simulink model "Kalman_filter"  (R2019b)
settings: Solver=FixedStepAuto  StartTime=0.0  StopTime=10.0  FixedStep=20e-3  RelTol=1e-3
values from neighbouring files (symbols this model uses):
  C = [0, 1]    [model_parameters.m]
undefined symbols (not defined in the file or in its folder): B_d, F, Q, R
settings Model: Creator=Олег  LastModifiedBy=Олег

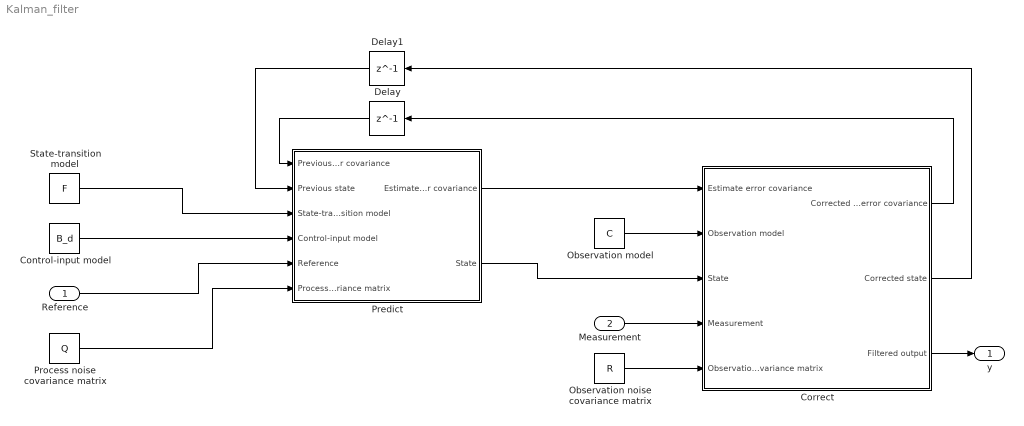
== system Kalman_filter ==
  Reference : Inport  PortDimensions=2
  Measurement : Inport  Port=2  PortDimensions=2
  Control-input model : Constant  Value=B_d
  Correct : Subsystem
  Delay : Delay  DelayLength=1  InitialCondition=eye(4)
  Delay1 : Delay  DelayLength=1  InitialCondition=zeros(4,1)
  Observation model : Constant  Value=C
  Observation noise covariance matrix : Constant  Value=R
  Predict : Subsystem
  Process noise covariance matrix : Constant  Value=Q
  State-transition model : Constant  Value=F
  y : Outport
  wires:
  State-transition model/1 -> Predict/3(State-transition model)
  Control-input model/1 -> Predict/4(Control-input model)
  Reference/1 -> Predict/5(Reference)
  Process noise covariance matrix/1 -> Predict/6(Process noise covariance matrix)
  Predict/2(State) -> Correct/3(State)
  Delay/1 -> Predict/1(Previous estimate error covariance)
  Delay1/1 -> Predict/2(Previous state)
  Predict/1(Estimate error covariance) -> Correct/1(Estimate error covariance)
  Observation model/1 -> Correct/2(Observation model)
  Measurement/1 -> Correct/4(Measurement)
  Observation noise covariance matrix/1 -> Correct/5(Observation noise covariance matrix)
  Correct/1(Corrected estimate error covariance) -> Delay/1
  Correct/2(Corrected state) -> Delay1/1
  Correct/3(Filtered output) -> y/1

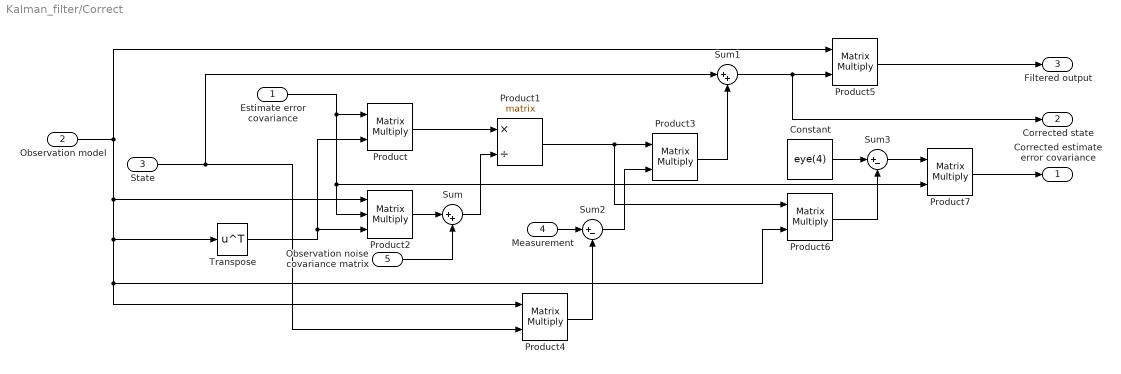
== system Kalman_filter/Correct ==
  Estimate error covariance : Inport
  Observation model : Inport  Port=2
  State : Inport  Port=3
  Measurement : Inport  Port=4
  Observation noise covariance matrix : Inport  Port=5
  Constant : Constant  Value=eye(4)
  Product{,3..7} (6 alike) : Product  Multiplication=Matrix(*)
  Product1 : Product  Inputs=*/  Multiplication=Matrix(*)
  Product2 : Product  Inputs=3  Multiplication=Matrix(*)
  Sum : Sum  Inputs=|++
  Sum1 : Sum  Inputs=|++
  Sum2 : Sum  Inputs=|+-
  Sum3 : Sum  Inputs=|+-
  Transpose : Math  Operator=transpose  SignedPower=off  SaturateOnIntegerOverflow=on
  Corrected estimate error covariance : Outport
  Corrected state : Outport  Port=2
  Filtered output : Outport  Port=3
  wires:
  Product3/1 -> Sum1/2
  Observation model/1 -> Product5/1, Product2/1, Transpose/1, Product6/2, Product4/1
  State/1 -> Product4/2, Sum1/1
  Sum1/1 -> Corrected state/1, Product5/2
  Product1/1 -> Product6/1, Product3/1
  Sum/1 -> Product1/2
  Product6/1 -> Sum3/2
  Estimate error covariance/1 -> Product/1, Product7/2, Product2/2
  Transpose/1 -> Product2/3, Product/2
  Sum3/1 -> Product7/1
  Sum2/1 -> Product3/2
  Product/1 -> Product1/1
  Constant/1 -> Sum3/1
  Product2/1 -> Sum/1
  Observation noise covariance matrix/1 -> Sum/2
  Product4/1 -> Sum2/2
  Measurement/1 -> Sum2/1
  Product7/1 -> Corrected estimate error covariance/1
  Product5/1 -> Filtered output/1

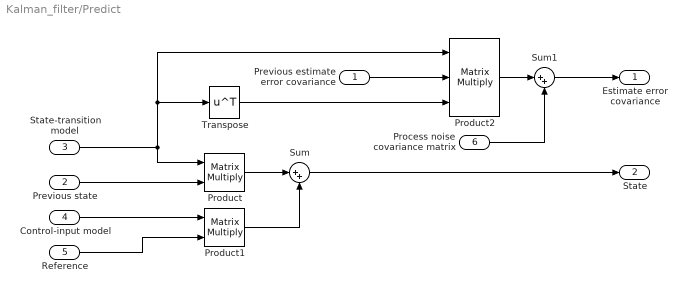
== system Kalman_filter/Predict ==
  Previous estimate error covariance : Inport
  Previous state : Inport  Port=2
  State-transition model : Inport  Port=3
  Control-input model : Inport  Port=4
  Reference : Inport  Port=5
  Process noise covariance matrix : Inport  Port=6
  Product : Product  Multiplication=Matrix(*)
  Product1 : Product  Multiplication=Matrix(*)
  Product2 : Product  Inputs=3  Multiplication=Matrix(*)
  Sum : Sum  Inputs=|++
  Sum1 : Sum  Inputs=|++
  Transpose : Math  Operator=transpose  SignedPower=off  SaturateOnIntegerOverflow=on
  Estimate error covariance : Outport
  State : Outport  Port=2
  wires:
  Control-input model/1 -> Product1/1
  Reference/1 -> Product1/2
  Product2/1 -> Sum1/1
  Transpose/1 -> Product2/3
  Product1/1 -> Sum/2
  Product/1 -> Sum/1
  Previous estimate error covariance/1 -> Product2/2
  State-transition model/1 -> Product/1, Transpose/1, Product2/1
  Process noise covariance matrix/1 -> Sum1/2
  Sum/1 -> State/1
  Sum1/1 -> Estimate error covariance/1
  Previous state/1 -> Product/2
